simulink model "CLab1_feedback"  (R2019a)
settings: Solver=VariableStepAuto  StartTime=0.0  StopTime=200  RelTol=1e-9
values from neighbouring files (symbols this model uses):
  D = 1    [CLab1.m]
  g = 1    [CLab1.m]
  k1 = .01    (= 0.01)    [CLab1.m]
  k2 = [.1*k1, 1*k1, 10*k1, 100*k1]    [CLab1.m]
  r = 0    [CLab1.m]
settings Model: Creator=Pranav Maddula  LastModifiedBy=Pranav Maddula

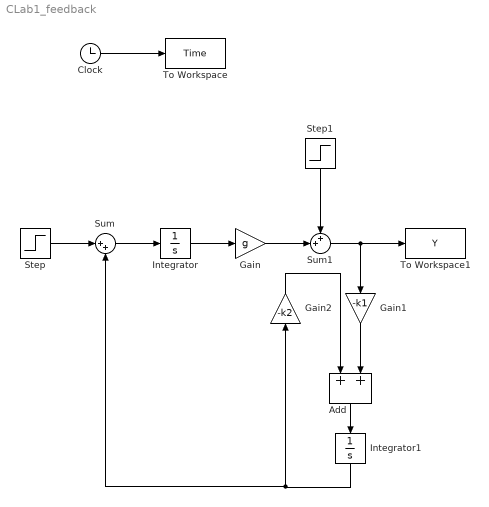
== system CLab1_feedback ==
  Add : Sum
  Clock : Clock
  Gain : Gain  Gain=g
  Gain1 : Gain  Gain=-k1
  Gain2 : Gain  Gain=-k2
  Integrator : Integrator
  Integrator1 : Integrator
  Step : Step  After=r  SampleTime=0
  Step1 : Step  After=D  SampleTime=0
  Sum : Sum  Inputs=|++
  Sum1 : Sum  Inputs=++|
  To Workspace : ToWorkspace  VariableName=Time  SampleTime=-1
  To Workspace1 : ToWorkspace  VariableName=Y  SampleTime=-1
  wires:
  Clock/1 -> To Workspace/1
  Sum/1 -> Integrator/1
  Integrator/1 -> Gain/1
  Gain/1 -> Sum1/2
  Step/1 -> Sum/1
  Sum1/1 -> Gain1/1, To Workspace1/1
  Gain1/1 -> Add/2
  Add/1 -> Integrator1/1
  Gain2/1 -> Add/1
  Integrator1/1 -> Sum/2, Gain2/1
  Step1/1 -> Sum1/1
